simulink model "math_rem_mod"  (Simulink 6.6)
settings: Solver=FixedStepDiscrete  StartTime=0.0  StopTime=10.0  FixedStep=1  RelTol=1e-3
settings Model: Creator=ksmyth  LastModifiedBy=ksmyth

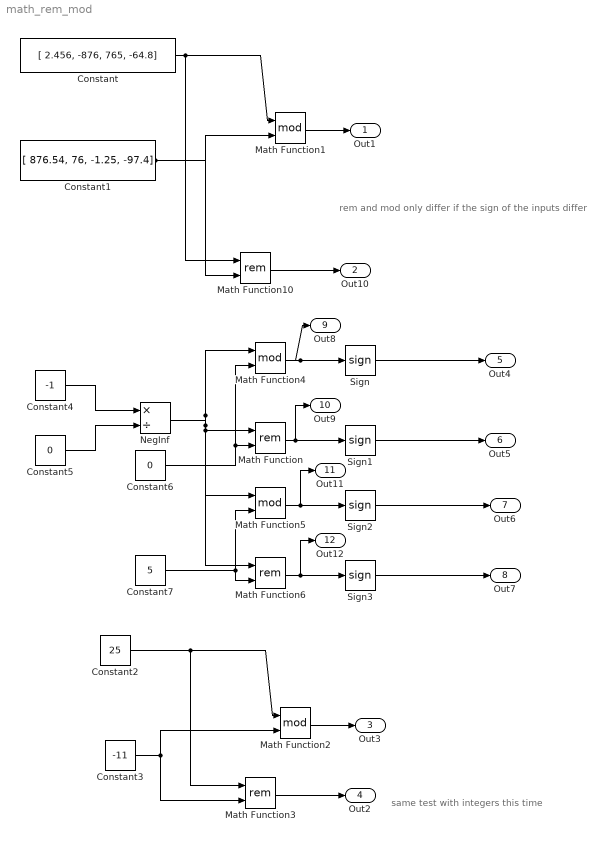
== system math_rem_mod ==
  note: rem and mod only differ if the sign of the inputs differ
  note: same test with integers this time
  Constant : Constant  Value=[ 2.456, -876, 765, -64.8]
  Constant1 : Constant  Value=[ 876.54, 76, -1.25, -97.4]
  Constant2 : Constant  Value=25
  Constant3 : Constant  Value=-11
  Constant4 : Constant  Value=-1
  Constant5 : Constant  Value=0
  Constant6 : Constant  Value=0
  Constant7 : Constant  Value=5
  Math Function{,3,6,10} (4 alike) : Math  Operator=rem  SaturateOnIntegerOverflow=on
  Math Function{1..2,4..5} (4 alike) : Math  Operator=mod  SaturateOnIntegerOverflow=on
  NegInf : Product  Inputs=*/  RndMeth=Zero
  Sign{,1..3} (4 alike) : Signum
  Out1 : Outport
  Out10 : Outport  Port=2
  Out3 : Outport  Port=3
  Out2 : Outport  Port=4
  Out4 : Outport  Port=5
  Out5 : Outport  Port=6
  Out6 : Outport  Port=7
  Out7 : Outport  Port=8
  Out8 : Outport  Port=9
  Out9 : Outport  Port=10
  Out11 : Outport  Port=11
  Out12 : Outport  Port=12
  wires:
  Constant/1 -> Math Function10/1, Math Function1/1
  Constant1/1 -> Math Function10/2, Math Function1/2
  Math Function10/1 -> Out10/1
  Math Function1/1 -> Out1/1
  Constant2/1 -> Math Function3/1, Math Function2/1
  Constant3/1 -> Math Function3/2, Math Function2/2
  Math Function3/1 -> Out2/1
  Math Function2/1 -> Out3/1
  Constant4/1 -> NegInf/1
  Constant5/1 -> NegInf/2
  NegInf/1 -> Math Function4/1, Math Function/1, Math Function5/1, Math Function6/1
  Constant6/1 -> Math Function4/2, Math Function/2
  Constant7/1 -> Math Function5/2, Math Function6/2
  Math Function4/1 -> Sign/1, Out8/1
  Sign/1 -> Out4/1
  Math Function/1 -> Sign1/1, Out9/1
  Sign1/1 -> Out5/1
  Math Function5/1 -> Sign2/1, Out11/1
  Sign2/1 -> Out6/1
  Math Function6/1 -> Sign3/1, Out12/1
  Sign3/1 -> Out7/1
